simulink model "threeDiskOscillatorRig_Q3_experiment"  (R2020a)
settings: Solver=VariableStepAuto  StartTime=0.0  StopTime=simTime  RelTol=1e-8
values from neighbouring files (symbols this model uses):
  den12 = [1 -1.94399066511 0.945546479969]    [Residual_generatorsQ2.mat]    (also in threeDiskOscillator_Q8.m = cell2mat(den1(2)); threeDiskOscillator_simData.m = cell2mat(den1(2)))
  den13 = [1 -1.94399066511 0.945546479969]    [Residual_generatorsQ2.mat]    (also in threeDiskOscillator_Q8.m = cell2mat(den1(3)); threeDiskOscillator_simData.m = cell2mat(den1(3)))
  den14 = [1 -1.94399066511 0.945546479969]    [Residual_generatorsQ2.mat]    (also in threeDiskOscillator_Q8.m = cell2mat(den1(4)); threeDiskOscillator_simData.m = cell2mat(den1(4)))
  den15 = [1 -1.94399066511 0.945546479969]    [Residual_generatorsQ2.mat]    (also in threeDiskOscillator_Q8.m = cell2mat(den1(5)); threeDiskOscillator_simData.m = cell2mat(den1(5)))
  den24 = [1 -1.94399066511 0.945546479969]    [Residual_generatorsQ2.mat]    (also in threeDiskOscillator_Q8.m = cell2mat(den2(4)); threeDiskOscillator_simData.m = cell2mat(den2(4)))
  den25 = [1 -1.94399066511 0.945546479969]    [Residual_generatorsQ2.mat]    (also in threeDiskOscillator_Q8.m = cell2mat(den2(5)); threeDiskOscillator_simData.m = cell2mat(den2(5)))
  J_2 = 0.00182883419357    [ECP_values_final.mat]    (also in Q2-5.mat; Residual_generators.mat; Residual_generatorsQ2.mat; threeDiskOscillator_ALL.m = ECP_values(2))
  J_3 = 0.00182883419357    [ECP_values_final.mat]    (also in Q2-5.mat; Residual_generators.mat; Residual_generatorsQ2.mat; threeDiskOscillator_ALL.m = ECP_values(3))
  k_1 = 2.78736928639    [ECP_values_final.mat]    (also in Q2-5.mat; Residual_generators.mat; Residual_generatorsQ2.mat; threeDiskOscillator_ALL.m = ECP_values(4))
  k_2 = 2.53389832968    [ECP_values_final.mat]    (also in Q2-5.mat; Residual_generators.mat; Residual_generatorsQ2.mat; threeDiskOscillator_ALL.m = ECP_values(5))
  num12 = [0.212678500804 0.425357001609 0.212678500804]    [Residual_generatorsQ2.mat]    (also in threeDiskOscillator_Q8.m = cell2mat(num1(2)); threeDiskOscillator_simData.m = cell2mat(num1(2)))
  num13 = [0.592813521017 1.18562704203 0.592813521017]    [Residual_generatorsQ2.mat]    (also in threeDiskOscillator_Q8.m = cell2mat(num1(3)); threeDiskOscillator_simData.m = cell2mat(num1(3)))
  num14 = [-98.3875982708 192.213418816 -98.3526974211]    [Residual_generatorsQ2.mat]    (also in threeDiskOscillator_Q8.m = cell2mat(num1(4)); threeDiskOscillator_simData.m = cell2mat(num1(4)))
  num15 = [0.538905697947 1.07781139589 0.538905697947]    [Residual_generatorsQ2.mat]    (also in threeDiskOscillator_Q8.m = cell2mat(num1(5)); threeDiskOscillator_simData.m = cell2mat(num1(5)))
  num24 = [0.538905697947 1.07781139589 0.538905697947]    [Residual_generatorsQ2.mat]    (also in threeDiskOscillator_Q8.m = cell2mat(num2(4)); threeDiskOscillator_simData.m = cell2mat(num2(4)))
  num25 = [-97.7963881502 193.399045858 -97.7582804996]    [Residual_generatorsQ2.mat]    (also in threeDiskOscillator_Q8.m = cell2mat(num2(5)); threeDiskOscillator_simData.m = cell2mat(num2(5)))
  T_s = 0.004    [ECP_values_final.mat]    (also in Q2-5.mat; Residual_generators.mat; Residual_generatorsQ2.mat; threeDiskOscillator_ALL.m)
settings Model: Creator=dimpa  LastModifiedBy=Administrator
settings DataIOCC: ReturnWorkspaceOutputs=off
settings DebuggingCC: ArithmeticOperatorsInVariantConditions=warning
settings SFSimCC: SimUseLocalCustomCode=off  CustomCodeUndefinedFunction=UseInterfaceOnly
settings RTWCC: RTWUseLocalCustomCode=off

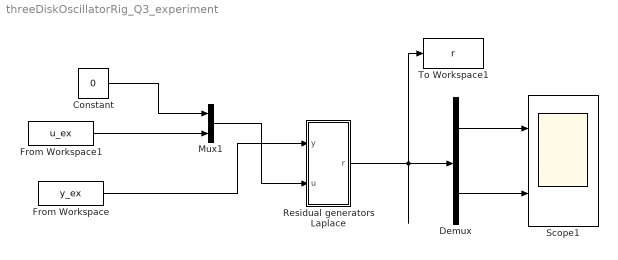
== system threeDiskOscillatorRig_Q3_experiment ==
  Constant : Constant  Value=0
  Demux : Demux  Outputs=2
  From Workspace : FromWorkspace  VariableName=y_ex  SampleTime=T_s
  From Workspace1 : FromWorkspace  VariableName=u_ex  SampleTime=T_s
  Mux1 : Mux  Inputs=2
  Residual generators Laplace : Subsystem
  Scope1 : Scope  NumInputPorts=2
  To Workspace1 : ToWorkspace  VariableName=r  SaveFormat=Timeseries  SampleTime=T_s
  wires:
  Residual generators Laplace/1(r) -> Demux/1, To Workspace1/1
  Demux/1 -> Scope1/1
  Demux/2 -> Scope1/2
  From Workspace1/1 -> Mux1/2
  Mux1/1 -> Residual generators Laplace/2(u)
  From Workspace/1 -> Residual generators Laplace/1(y)
  Constant/1 -> Mux1/1

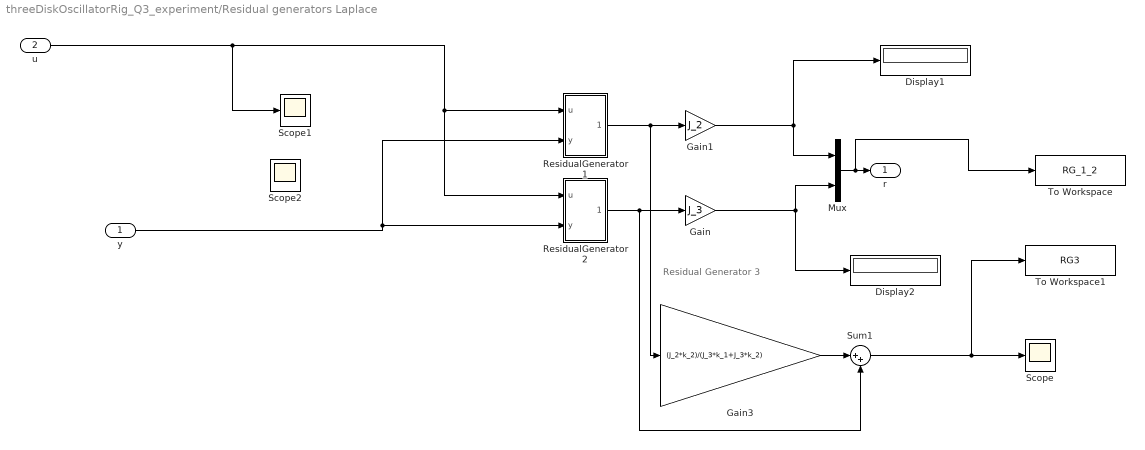
== system threeDiskOscillatorRig_Q3_experiment/Residual generators Laplace ==
  note: Residual Generator 3
  y : Inport
  u : Inport  Port=2
  Display1 : Display
  Display2 : Display
  Gain : Gain  Gain=J_3
  Gain1 : Gain  Gain=J_2
  Gain3 : Gain  Gain=(J_2*k_2)/(J_3*k_1+J_3*k_2)
  Mux : Mux  Inputs=2
  ResidualGenerator 1 : Subsystem
  ResidualGenerator 2 : Subsystem
  Scope : Scope
  Scope1 : Scope
  Scope2 : Scope
  Sum1 : Sum  Inputs=|++
  To Workspace : ToWorkspace  VariableName=RG_1_2  SaveFormat=Timeseries  SampleTime=-1
  To Workspace1 : ToWorkspace  VariableName=RG3  SaveFormat=Timeseries  SampleTime=-1
  r : Outport  VectorParamsAs1DForOutWhenUnconnected=off
  wires:
  Mux/1 -> To Workspace/1, r/1
  ResidualGenerator 2/1(Out1) -> Gain/1, Sum1/2
  Sum1/1 -> To Workspace1/1, Scope/1
  Gain3/1 -> Sum1/1
  ResidualGenerator 1/1(Out1) -> Gain1/1, Gain3/1
  Gain/1 -> Mux/2, Display2/1
  u/1 -> ResidualGenerator 2/1(u), ResidualGenerator 1/1(u), Scope1/1
  y/1 -> ResidualGenerator 2/2(y), ResidualGenerator 1/2(y)
  Gain1/1 -> Display1/1, Mux/1

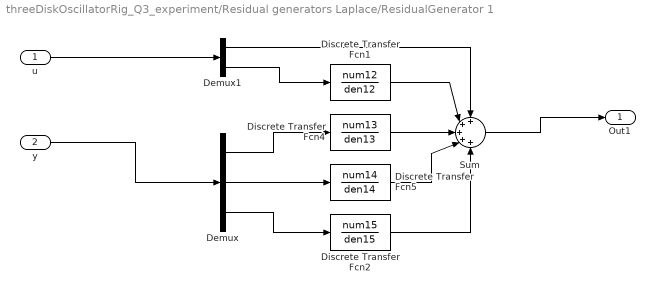
== system threeDiskOscillatorRig_Q3_experiment/Residual generators Laplace/ResidualGenerator 1 ==
  u : Inport
  y : Inport  Port=2
  Demux : Demux  Outputs=3
  Demux1 : Demux  Outputs=2
  Discrete Transfer Fcn1 : DiscreteTransferFcn  Numerator=num12  Denominator=den12
  Discrete Transfer Fcn2 : DiscreteTransferFcn  Numerator=num15  Denominator=den15
  Discrete Transfer Fcn4 : DiscreteTransferFcn  Numerator=num13  Denominator=den13
  Discrete Transfer Fcn5 : DiscreteTransferFcn  Numerator=num14  Denominator=den14
  Sum : Sum  Inputs=+++++
  Out1 : Outport
  wires:
  Demux/2 -> Discrete Transfer Fcn5/1
  Discrete Transfer Fcn5/1 -> Sum/4
  Sum/1 -> Out1/1
  Demux/1 -> Discrete Transfer Fcn4/1
  Demux/3 -> Discrete Transfer Fcn2/1
  Discrete Transfer Fcn1/1 -> Sum/2
  Discrete Transfer Fcn4/1 -> Sum/3
  Demux1/2 -> Discrete Transfer Fcn1/1
  Discrete Transfer Fcn2/1 -> Sum/5
  y/1 -> Demux/1
  u/1 -> Demux1/1
  Demux1/1 -> Sum/1

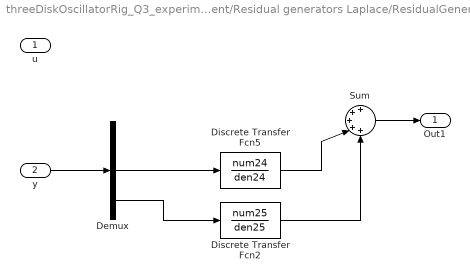
== system threeDiskOscillatorRig_Q3_experiment/Residual generators Laplace/ResidualGenerator 2 ==
  u : Inport
  y : Inport  Port=2
  Demux : Demux  Outputs=3
  Discrete Transfer Fcn2 : DiscreteTransferFcn  Numerator=num25  Denominator=den25
  Discrete Transfer Fcn5 : DiscreteTransferFcn  Numerator=num24  Denominator=den24
  Sum : Sum  Inputs=+++++
  Out1 : Outport
  wires:
  Demux/2 -> Discrete Transfer Fcn5/1
  Discrete Transfer Fcn5/1 -> Sum/4
  Sum/1 -> Out1/1
  Demux/3 -> Discrete Transfer Fcn2/1
  Discrete Transfer Fcn2/1 -> Sum/5
  y/1 -> Demux/1
